simulink model "FlowControllerPrototyping"  (R2021a)
settings: Solver=VariableStepAuto  StartTime=0.0  StopTime=4  RelTol=1e-3
libraries: EdgesLibrary x8, StreetLanesLibrary x6, SourcesAndSinksLibrary x4
(part 1 of 2)
settings Model: Creator=phill  LastModifiedBy=phill

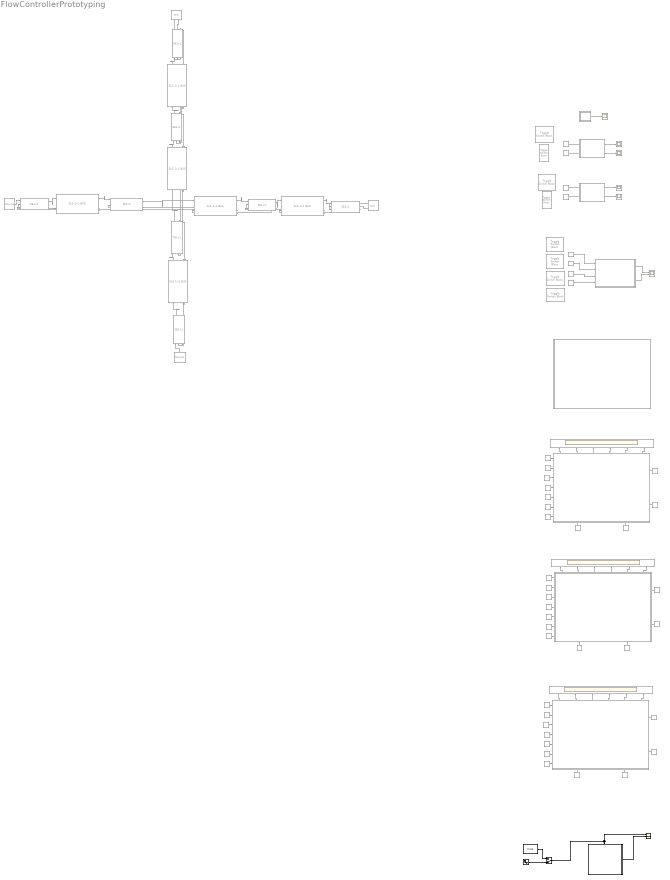
== system FlowControllerPrototyping ==
  note: Test if we can use input events to activate our controllers only if some of the inputs change. Result: Regardless of what the input event is set to (rising/falling/both), it CONSISTENTLY misses to trigger on the first of the afronementioned occurences
  note: does not work completely
  note: Just view a conflict based purely on signal strength ("car is waiting at signalX"),
      | without asking for the filling state of cross-section-segments. In this case
      | signal1 has priority before signal2
  note: Test: see how we can execute multiple transitions inside the chart during a single outer simulation step. seems to work if we chain the transitions after another using junctions
  note: does not work completely
  note: does not work completely
  note: seems to work
  Ali : Constant  Commented=on
  Ali Bo : Constant  Commented=on  Value=0
  Ali Bo1 : Constant  Commented=on  Value=0
  Ali Bo2 : Constant  Commented=on  Value=0
  Ali1 : Constant  Commented=on
  Ali2 : Constant  Commented=on
  Ari : Constant  Commented=on
  Ari Co : Constant  Commented=on  Value=0
  Ari Co1 : Constant  Commented=on  Value=0
  Ari Co2 : Constant  Commented=on  Value=0
  Ari1 : Constant  Commented=on
  Ari2 : Constant  Commented=on
  Brs : Constant  Commented=on
  Brs Ao : Constant  Commented=on  Value=0
  Brs Ao1 : Constant  Commented=on  Value=0
  Brs Ao2 : Constant  Commented=on  Value=0
  Brs Co : Constant  Commented=on
  Brs Co1 : Constant  Commented=on  Value=0
  Brs Co2 : Constant  Commented=on  Value=0
  Brs1 : Constant  Commented=on  Value=0
  Brs2 : Constant  Commented=on  Value=0
  Chart : Stateflow chart  Commented=on  TreatAsAtomicUnit=on
  Chart1 : Stateflow chart  Commented=on  TreatAsAtomicUnit=on
      settings: PortSchema="{\"entries\":[{\"content\":{\"sides\":[{\"content\":{\"connectorIds\":[\"In6\",\"In7\",\"In8\",\"In9\",\"In10\",\"In11\",\"In5\"]},\"type\":\"ConnectorPlacement.EquallySpacedRectSide\",\"uuid\":\"dee1a780-e9dd-4205-adb9-3e9cb1ec0cd6\"},{\"content\":{\"connectorIds\":[\"In4\",\"In3\"],\"side\":\"RIGHT\"},\"type\":\"ConnectorPlacement.EquallySpacedRectSide\",\"uuid\":\"bc6af08d-2df8-4a74-93d0-032b7c1c381c\"},{\"content\":{\"connectorIds\":[\"Out5\",\"Out6\",\"Out1\",\"Out2\",\"Out3\",\"Out4\"],\"side\":\"TOP\"},\"type\":\"ConnectorPlacement.EquallySpacedRectSide\",\"uuid\":\"98fea325-c9fc-472d-8e1a-d846d6e99e12\"},{\"content\":{\"connectorIds\":[\"In1\",\"In2\"],\"side\":\"BOTTOM\"},\"type\":\"ConnectorPlacement.EquallySpacedRectSide\",\"uuid\":\"a092283f-ef46-48e2-a5f8-8210ac00b2f9\"}]},\"type\":\"ConnectorPlacement.EquallySpacedConnector\",\"uuid\":\"33a851aa-4180-41c0-b4bb-9b9c3be41936\"}],\"packageUris\":[\"http://schema.mathworks.com/mf0/Connector/R2020b\"],\"version\":\"1.0\"}"
  Chart2 : Stateflow chart  Commented=on  TreatAsAtomicUnit=on
      settings: PortSchema="{\"entries\":[{\"content\":{\"sides\":[{\"content\":{\"connectorIds\":[\"In6\",\"In7\",\"In8\",\"In9\",\"In10\",\"In11\",\"In5\"]},\"type\":\"ConnectorPlacement.EquallySpacedRectSide\",\"uuid\":\"dee1a780-e9dd-4205-adb9-3e9cb1ec0cd6\"},{\"content\":{\"connectorIds\":[\"In4\",\"In3\"],\"side\":\"RIGHT\"},\"type\":\"ConnectorPlacement.EquallySpacedRectSide\",\"uuid\":\"bc6af08d-2df8-4a74-93d0-032b7c1c381c\"},{\"content\":{\"connectorIds\":[\"Out5\",\"Out6\",\"Out1\",\"Out2\",\"Out3\",\"Out4\"],\"side\":\"TOP\"},\"type\":\"ConnectorPlacement.EquallySpacedRectSide\",\"uuid\":\"98fea325-c9fc-472d-8e1a-d846d6e99e12\"},{\"content\":{\"connectorIds\":[\"In1\",\"In2\"],\"side\":\"BOTTOM\"},\"type\":\"ConnectorPlacement.EquallySpacedRectSide\",\"uuid\":\"a092283f-ef46-48e2-a5f8-8210ac00b2f9\"}]},\"type\":\"ConnectorPlacement.EquallySpacedConnector\",\"uuid\":\"33a851aa-4180-41c0-b4bb-9b9c3be41936\"}],\"packageUris\":[\"http://schema.mathworks.com/mf0/Connector/R2020b\"],\"version\":\"1.0\"}"
  Chart3 : Stateflow chart  Commented=on  TreatAsAtomicUnit=on
      settings: PortSchema="{\"entries\":[{\"content\":{\"sides\":[{\"content\":{\"connectorIds\":[\"In6\",\"In7\",\"In8\",\"In9\",\"In10\",\"In11\",\"In5\"]},\"type\":\"ConnectorPlacement.EquallySpacedRectSide\",\"uuid\":\"dee1a780-e9dd-4205-adb9-3e9cb1ec0cd6\"},{\"content\":{\"connectorIds\":[\"In4\",\"In3\"],\"side\":\"RIGHT\"},\"type\":\"ConnectorPlacement.EquallySpacedRectSide\",\"uuid\":\"bc6af08d-2df8-4a74-93d0-032b7c1c381c\"},{\"content\":{\"connectorIds\":[\"Out5\",\"Out6\",\"Out1\",\"Out2\",\"Out3\",\"Out4\"],\"side\":\"TOP\"},\"type\":\"ConnectorPlacement.EquallySpacedRectSide\",\"uuid\":\"98fea325-c9fc-472d-8e1a-d846d6e99e12\"},{\"content\":{\"connectorIds\":[\"In1\",\"In2\"],\"side\":\"BOTTOM\"},\"type\":\"ConnectorPlacement.EquallySpacedRectSide\",\"uuid\":\"a092283f-ef46-48e2-a5f8-8210ac00b2f9\"}]},\"type\":\"ConnectorPlacement.EquallySpacedConnector\",\"uuid\":\"33a851aa-4180-41c0-b4bb-9b9c3be41936\"}],\"packageUris\":[\"http://schema.mathworks.com/mf0/Connector/R2020b\"],\"version\":\"1.0\"}"
  Chart4 : Stateflow chart  Commented=on  TreatAsAtomicUnit=on
      settings: PortSchema="{\"entries\":[{\"content\":{\"sides\":[{\"content\":{\"connectorIds\":[\"In6\",\"In7\",\"In8\",\"In9\",\"In10\",\"In11\",\"In5\"]},\"type\":\"ConnectorPlacement.EquallySpacedRectSide\",\"uuid\":\"dee1a780-e9dd-4205-adb9-3e9cb1ec0cd6\"},{\"content\":{\"connectorIds\":[\"In4\",\"In3\"],\"side\":\"RIGHT\"},\"type\":\"ConnectorPlacement.EquallySpacedRectSide\",\"uuid\":\"bc6af08d-2df8-4a74-93d0-032b7c1c381c\"},{\"content\":{\"connectorIds\":[\"Out5\",\"Out6\",\"Out1\",\"Out2\",\"Out3\",\"Out4\"],\"side\":\"TOP\"},\"type\":\"ConnectorPlacement.EquallySpacedRectSide\",\"uuid\":\"98fea325-c9fc-472d-8e1a-d846d6e99e12\"},{\"content\":{\"connectorIds\":[\"In1\",\"In2\"],\"side\":\"BOTTOM\"},\"type\":\"ConnectorPlacement.EquallySpacedRectSide\",\"uuid\":\"a092283f-ef46-48e2-a5f8-8210ac00b2f9\"}]},\"type\":\"ConnectorPlacement.EquallySpacedConnector\",\"uuid\":\"33a851aa-4180-41c0-b4bb-9b9c3be41936\"}],\"packageUris\":[\"http://schema.mathworks.com/mf0/Connector/R2020b\"],\"version\":\"1.0\"}"
  Cl : Constant  Commented=on
  Cl Ao : Constant  Commented=on  Value=0
  Cl Ao1 : Constant  Commented=on  Value=0
  Cl Ao2 : Constant  Commented=on  Value=0
  Cl1 : Constant  Commented=on
  Cl2 : Constant  Commented=on
  Cs : Constant  Commented=on  Value=0
  Cs Bo : Constant  Commented=on  Value=0
  Cs Bo1 : Constant  Commented=on  Value=0
  Cs Bo2 : Constant  Commented=on  Value=0
  Cs1 : Constant  Commented=on  Value=0
  Cs2 : Constant  Commented=on  Value=0
  Manual Switch : ManualSwitch  CurrentSetting=0
  Pulse Generator : DiscretePulseGenerator  PulseType=Time based  Period=1  PulseWidth=50  PhaseDelay=1
  SE1x{1..6} (6 alike) : EdgesLibrary/SE1x1  Commented=on  Rk=1
  SLS 1x1 BUS{,1..5} (6 alike) : StreetLanesLibrary/SLS 1x1 BUS  Commented=on  Kz=3  Tz=1
  Scope{,1..4} (5 alike) : Scope  Commented=on
  Scope5 : Scope  Commented=on  NumInputPorts=2
  Scope6 : Scope  Commented=on  NumInputPorts=6
  Scope7 : Scope  Commented=on  NumInputPorts=6
  Scope8 : Scope  Commented=on  NumInputPorts=6
  Scope9 : Scope  NumInputPorts=2
  SimpleFlowController : Stateflow chart  Commented=on  TreatAsAtomicUnit=on
  Sine Wave : Sin  SampleTime=0
  Sink : SourcesAndSinksLibrary/Sink  Commented=on  SystemSampleTime=-1  VariantActivationTime=update diagram  Latency=0  AutoFrameSizeCalculation=off
      settings: PortSchema="{\"entries\":[{\"content\":{\"sides\":[{\"content\":{\"connectorIds\":[\"Out1\",\"Out2\"]},\"type\":\"ConnectorPlacement.EquallySpacedRectSide\",\"uuid\":\"9fd2383e-3590-4f0f-bafc-5a4adfbb32b4\"},{\"content\":{\"connectorIds\":[],\"side\":\"RIGHT\"},\"type\":\"ConnectorPlacement.EquallySpacedRectSide\",\"uuid\":\"1e687aa9-1098-45bd-a1f6-ea403f3f2897\"},{\"content\":{\"connectorIds\":[],\"side\":\"TOP\"},\"type\":\"ConnectorPlacement.EquallySpacedRectSide\",\"uuid\":\"fe6eaa71-085c-414b-983a-a0e72e52a49c\"}]},\"type\":\"ConnectorPlacement.EquallySpacedConnector\",\"uuid\":\"370c1712-4373-4726-99c2-6cb04807ece1\"}],\"packageUris\":[\"http://schema.mathworks.com/mf0/Connector/R2020b\"],\"version\":\"1.0\"}"
  Sink1 : SourcesAndSinksLibrary/Sink  Commented=on  SystemSampleTime=-1  VariantActivationTime=update diagram  Latency=0  AutoFrameSizeCalculation=off
      settings: PortSchema="{\"entries\":[{\"content\":{\"sides\":[{\"content\":{\"connectorIds\":[\"Out1\",\"Out2\"]},\"type\":\"ConnectorPlacement.EquallySpacedRectSide\",\"uuid\":\"9fd2383e-3590-4f0f-bafc-5a4adfbb32b4\"},{\"content\":{\"connectorIds\":[],\"side\":\"RIGHT\"},\"type\":\"ConnectorPlacement.EquallySpacedRectSide\",\"uuid\":\"1e687aa9-1098-45bd-a1f6-ea403f3f2897\"},{\"content\":{\"connectorIds\":[],\"side\":\"TOP\"},\"type\":\"ConnectorPlacement.EquallySpacedRectSide\",\"uuid\":\"fe6eaa71-085c-414b-983a-a0e72e52a49c\"}]},\"type\":\"ConnectorPlacement.EquallySpacedConnector\",\"uuid\":\"370c1712-4373-4726-99c2-6cb04807ece1\"}],\"packageUris\":[\"http://schema.mathworks.com/mf0/Connector/R2020b\"],\"version\":\"1.0\"}"
  Source : SourcesAndSinksLibrary/Source  Commented=on  SystemSampleTime=-1  VariantActivationTime=update diagram  Latency=0  AutoFrameSizeCalculation=off
  Source1 : SourcesAndSinksLibrary/Source  Commented=on  SystemSampleTime=-1  VariantActivationTime=update diagram  Latency=0  AutoFrameSizeCalculation=off
  TE1x1 : EdgesLibrary/TE1x1  Commented=on  Rk=1
  TE1x2 : EdgesLibrary/TE1x1  Commented=on  Rk=1
  Testchart : Stateflow chart  TreatAsAtomicUnit=on
  Toggle Switch{,1..7} (8 alike) : ToggleSwitchBlock  Commented=on
      settings: Values={{'Off', 'On'}, [0 1]}
  innerBT : Constant  Commented=on  Value=0
  innerLR : Constant  Commented=on  Value=0
  mincontroller_pseudoparallel : Stateflow chart  Commented=on  TreatAsAtomicUnit=on
  mincontroller_sequential : Stateflow chart  Commented=on  TreatAsAtomicUnit=on
  x01 : Constant  Commented=on
  x02 : Constant  Commented=on
  x0Bottom : Constant  Commented=on
  x0Left : Constant  Commented=on
  x0a : Constant  Commented=on
  x0b : Constant  Commented=on
  wires:
  Source/1 -> SE1x4/1
  SLS 1x1 BUS/6 -> SE1x4/2
  SLS 1x1 BUS/7 -> SE1x4/3
  SE1x4/1 -> SLS 1x1 BUS/1
  SLS 1x1 BUS/2 -> TE1x1/1
  TE1x1/2 -> SLS 1x1 BUS/2
  SLS 1x1 BUS1/6 -> TE1x1/3
  SLS 1x1 BUS1/7 -> TE1x1/4
  TE1x1/1 -> SLS 1x1 BUS1/1
  SLS 1x1 BUS1/2 -> SE1x1/1
  SE1x1/2 -> SLS 1x1 BUS1/2
  SLS 1x1 BUS2/6 -> SE1x1/2
  SLS 1x1 BUS2/7 -> SE1x1/3
  SE1x1/1 -> SLS 1x1 BUS2/1
  SLS 1x1 BUS2/2 -> SE1x3/1
  SE1x3/2 -> SLS 1x1 BUS2/2
  Sink/1 -> SE1x3/2
  Sink/2 -> SE1x3/3
  Source1/1 -> SE1x5/1
  SE1x5/1 -> SLS 1x1 BUS3/1
  SLS 1x1 BUS3/6 -> SE1x5/2
  SLS 1x1 BUS3/7 -> SE1x5/3
  TE1x2/2 -> SLS 1x1 BUS3/2
  SLS 1x1 BUS3/2 -> TE1x2/1
  TE1x2/1 -> SLS 1x1 BUS4/1
  SLS 1x1 BUS4/7 -> TE1x2/4
  SLS 1x1 BUS4/6 -> TE1x2/3
  SE1x2/2 -> SLS 1x1 BUS4/2
  SLS 1x1 BUS4/2 -> SE1x2/1
  SE1x2/1 -> SLS 1x1 BUS5/1
  SLS 1x1 BUS5/7 -> SE1x2/3
  SLS 1x1 BUS5/6 -> SE1x2/2
  SE1x6/2 -> SLS 1x1 BUS5/2
  SLS 1x1 BUS5/2 -> SE1x6/1
  Sink1/1 -> SE1x6/2
  Sink1/2 -> SE1x6/3
  Chart/1(y) -> Scope/1
  x01/1 -> mincontroller_pseudoparallel/1(signal1)
  x02/1 -> mincontroller_pseudoparallel/2(signal2)
  mincontroller_pseudoparallel/1(enable1) -> Scope1/1
  mincontroller_pseudoparallel/2(enable2) -> Scope2/1
  mincontroller_sequential/1(enable1) -> Scope3/1
  mincontroller_sequential/2(enable2) -> Scope4/1
  x0a/1 -> mincontroller_sequential/1(signal1)
  x0b/1 -> mincontroller_sequential/2(signal2)
  x0Left/1 -> SimpleFlowController/1(x0Left)
  x0Bottom/1 -> SimpleFlowController/2(x0Bottom)
  innerLR/1 -> SimpleFlowController/3(innerLR)
  innerBT/1 -> SimpleFlowController/4(innerBT)
  SimpleFlowController/1(openLeft) -> Scope5/1
  SimpleFlowController/2(openBottom) -> Scope5/2
  Ali Bo/1 -> Chart2/6(Ali_Bo)
  Ari Co/1 -> Chart2/7(Ari_Co)
  Ali/1 -> Chart2/1(Ali)
  Ari/1 -> Chart2/2(Ari)
  Cl Ao/1 -> Chart2/8(Cl_Ao)
  Cs Bo/1 -> Chart2/9(Cs_Bo)
  Brs Co/1 -> Chart2/10(Brs_Co)
  Brs Ao/1 -> Chart2/11(Brs_Ao)
  Brs/1 -> Chart2/5(Brs)
  Chart2/5(enableBrs11) -> Scope6/1
  Chart2/6(enableBrs12) -> Scope6/2
  Chart2/1(enableAli3) -> Scope6/3
  Chart2/2(enableAri4) -> Scope6/4
  Chart2/3(enableCl7) -> Scope6/5
  Chart2/4(enableCs8) -> Scope6/6
  Cs/1 -> Chart2/4(Cs)
  Cl/1 -> Chart2/3(Cl)
  Cs1/1 -> Chart3/4(Cs)
  Cl1/1 -> Chart3/3(Cl)
  Cl Ao1/1 -> Chart3/8(Cl_Ao)
  Ari Co1/1 -> Chart3/7(Ari_Co)
  Chart3/2(enableAri4) -> Scope7/4
  Chart3/3(enableCl7) -> Scope7/5
  Ali Bo1/1 -> Chart3/6(Ali_Bo)
  Chart3/1(enableAli3) -> Scope7/3
  Chart3/6(enableBrs12) -> Scope7/2
  Cs Bo1/1 -> Chart3/9(Cs_Bo)
  Brs Co1/1 -> Chart3/10(Brs_Co)
  Chart3/4(enableCs8) -> Scope7/6
  Ali1/1 -> Chart3/1(Ali)
  Chart3/5(enableBrs11) -> Scope7/1
  Ari1/1 -> Chart3/2(Ari)
  Brs Ao1/1 -> Chart3/11(Brs_Ao)
  Brs1/1 -> Chart3/5(Brs)
  Brs2/1 -> Chart4/5(Brs)
  Chart4/3(enableCl7) -> Scope8/5
  Ali2/1 -> Chart4/1(Ali)
  Chart4/5(enableBrs11) -> Scope8/1
  Brs Ao2/1 -> Chart4/11(Brs_Ao)
  Chart4/6(enableBrs12) -> Scope8/2
  Cs Bo2/1 -> Chart4/9(Cs_Bo)
  Chart4/2(enableAri4) -> Scope8/4
  Chart4/4(enableCs8) -> Scope8/6
  Ari2/1 -> Chart4/2(Ari)
  Ali Bo2/1 -> Chart4/6(Ali_Bo)
  Cs2/1 -> Chart4/4(Cs)
  Ari Co2/1 -> Chart4/7(Ari_Co)
  Chart4/1(enableAli3) -> Scope8/3
  Cl Ao2/1 -> Chart4/8(Cl_Ao)
  Cl2/1 -> Chart4/3(Cl)
  Brs Co2/1 -> Chart4/10(Brs_Co)
  Manual Switch/1 -> Scope9/1, Testchart/Trigger
  Testchart/1(y) -> Scope9/2
  Sine Wave/1 -> Manual Switch/2
  Pulse Generator/1 -> Manual Switch/1

== stateflow chart FlowControllerPrototyping/SimpleFlowController ==
  state Initial
  note: Bottom
  note: Left
  (default) -> Initial : {openLeft = 0; openBottom = 0;}
  (junction 10) -> (junction 14) [order 1] : [x0Left > 0 && x0Bottom == 0 && innerBT == 0]{openLeft=1;}
  Initial -> (junction 10) [order 1] : [x0Bottom > 0 && innerLR == 0]{openBottom=1;}
  (junction 10) -> (junction 14) [order 2] : {openLeft=0;}
  Initial -> (junction 10) [order 2] : {openBottom=0;}
  (junction 14) -> (junction 15)
  (junction 15) -> Initial
  data: x0Left input; x0Bottom input; openLeft output; openBottom output; innerLR input; innerBT input

== stateflow chart FlowControllerPrototyping/mincontroller_sequential ==
  note: for signal 2
  note: for signal 1
  state Superstate
  (default) -> Superstate : {enable1 = 0; enable2 = 0}
  (junction 26) -> (junction 27) [order 1] : [signal2 > 0 && signal1 == 0]{enable2=1;}
  Superstate -> (junction 26) [order 1] : [signal1 > 0]{enable1 = 1;}
  Superstate -> (junction 26) [order 2] : {enable1=0;}
  (junction 26) -> (junction 27) [order 2] : {enable2=0;}
  (junction 27) -> (junction 34)
  (junction 34) -> Superstate
  data: enable1 output; enable2 output; signal1 input; signal2 input

== stateflow chart FlowControllerPrototyping/Chart1 ==
  note: Notizen (mal auf Deutsch):
      | wenn an einer kante etwas anliegt und keine der stärkeren kanten etwas anliegen hat,
      | 	und die konfliktbereiche frei sind: schalte kante frei
      | 	<Ali 3> wird dominiert von <Cl 7> und <Cs 8>  [Kreuzungen: <Brs Co> <Cl Ao> <Cs Bo>
      | 	<Ari 4> wird nicht dominiert [Kreuzungen: <Brs Co>
      | 	<Cl 7> wird dominiert von <Brs 11> und <Brs 12> [Kreuzungen: <Brs Co> <Brs Ao>
      | 	<Cs 8> wird nicht dominiert [Kreuzungen: <Ali Bo>
      | 	<Brs 11> wird dominiert von <Ali 3> und <Ari 4> [Kreuzungen: <Brs Ao> <Ali Bo> <Ari Co>
      | 	<Brs 12> wird nicht dominiert [Kreuzungen: <Cl Ao>
      |
      | 	Anmerkung: die einflüsse Brs11 und Brs12 behindern sich nicht. da beide kanten an
      | 	EIN UND DEMSELBEN SEGMENT liegen, und unsere 0.5:0.5 gewichtung schon suggeriert,
      | 	dass sich hier die autos "spalten", können sich die autos beim "Parallelen" fließen
      | 	in die segmente <Brs Co> und <Brs Ao> nicht wirklich in die quere kommen. Oder selbst wenn sie es
      |       tun, können wir nichts dagegen unternehmen - wenn wir einem der pfade gegenüber dem anderen
      | 	priorität geben, wird bei dem anderen jeweils NIE etwas fließen. Damit müssen wir wohl leben :(
      |
      | a)
      | [Ali > 0 && Cl == 0 && Cs == 0 && Brs_Co == 0 && Cl_Ao == 0 && Cs_Bo == 0]{enableAli3=1;}
      | else {enableAli3=0;}
      | b)
      | [Ari > 0 && Brs_Co == 0]{enableAri4=1;}
      | else {enableAri4=0;}
      | c)
      | [Cl > 0 && Brs == 0 && Brs_Co == 0 && Brs_Ao == 0]{enableCl7=1;}
      | else {enableCl7=0;}
      | d)
      | [Cs > 0 && Ali_Bo == 0]{enableCs8=1;}
      | else {enableCs8=0;}
      | e)
      | [Brs > 0 && Ali == 0 && Ari == 0 && Ali_Bo == 0 && Ari_Co == 0]{enableBrs11=1;}
      | else {enableBrs11=0;}
      | f)
      | [Brs > 0 && Cl_Ao == 0]{enableBrs12=1;}
      | else {enableBrs12=0;}
      |
      | Anmerkung: Da es im Falle [Ali > 0 && Brs > 0 && Cl > 0] einen deadlock gibt, müssen wir uns entscheiden, wer fahren darf. Da die "gerade" strecke vermutlich am ehesten einer hauptstraße
      | entsprechen würde, wird hier die regel so modifiziert, dass die von "unten" (Ali) kommenden autos
      | freiwillig auf Brs (und gezwungenermaßen auf Cl) warten, um stau auf der hauptstraße zu reduzieren.
      | Dazu erweitern wir die anliege-conditionen der Regel e) zu:
      | e')
      | [ ( (Brs > 0 && Ali == 0 && Ari == 0) || (Ali > 0 && Brs > 0 && Cl >0 && Ari == 0) ) && Ali_Bo == 0 && Ari_Co == 0]{enableBrs11=1;}
      | else {enableBrs11=0;} klappt nicht
      |
      | Somit verhält sich das T stück dann so, als würde magischerweise ein Vorfahrt achten schild
      | am unteren Eingang solange stehen, wie ein deadlock droht, und danach wieder verschwinden.
      | Unsere Autofahrer sind also sehr sozial unterwegs...
  note: ?
  state InitiatePerStepCheck
  note: Brs-11-<Brs Co>-6-Co
      | (Links will geradeaus)
  note: Brs-12-<Brs Ao>-1-Ao
      | (Links will geradeaus)
  note: Ari-4-<Ari Co>-5-Co
      | (Unten will rechts abbiegen)
  note: Cl-7-<Cl Ao>-2-Ao
      | (Rechts will links abbiegen)
  note: Cs-8-<Cl Ao>-9-Bo
      | (Rechts will geradeaus)
  note: Ali-3-<Ali Bo>-10-Bo
      | (Unten will Links abbiegen)
  note: Deadlock-Resolution
  InitiatePerStepCheck -> (junction 23) [order 1] : [Ali > 0 && Cl == 0 && Cs == 0 && Brs_Co == 0 && Cl_Ao == 0 && Cs_Bo == 0]
      | {enableAli3=1;}
  (junction 23) -> (junction 29) [order 1] : [Ari > 0 && Brs_Co == 0]{enableAri4=1;}
  (junction 29) -> (junction 36) [order 1] : [Cl > 0 && Brs == 0 && Brs_Co == 0 && Brs_Ao == 0]{enableCl7=1; }
  (junction 39) -> (junction 40) [order 1] : [  ( (Brs > 0 && Ali == 0 && Ari == 0) || (Ali > 0 && Brs > 0 && Cl > 0 && Ari == 0) ) && Ali_Bo == 0 && Ari_Co == 0]{enableBrs11=1;}
  (junction 40) -> (junction 45) [order 1] : [Brs > 0 && Cl_Ao == 0]{enableBrs12=1;}
  (junction 36) -> (junction 39) [order 1] : [Cs > 0 && Ali_Bo == 0]{enableCs8=1;}
  (junction 39) -> (junction 40) [order 2] : {enableBrs11=0;}
  (junction 29) -> (junction 36) [order 2] : {enableCl7=0;}
  (junction 36) -> (junction 39) [order 2] : {enableCs8=0;}
  (junction 23) -> (junction 29) [order 2] : {enableAri4=0;}
  (junction 40) -> (junction 45) [order 2] : {enableBrs12=0;}
  InitiatePerStepCheck -> (junction 23) [order 2] : {enableAli3=0;}
  (junction 45) -> (junction 53)
  (default) -> InitiatePerStepCheck : {enableAli3 = 0; enableAri4 = 0;
      | enableCl7 = 0; enableCs8 = 0;
      | enableBrs11 = 0; enableBrs12 = 0;}
  (junction 53) -> InitiatePerStepCheck
  data: Ali input; Ari input; Cl input; Cs input; Brs input; Ali_Bo input; Ari_Co input; Cl_Ao input; Cs_Bo input; Brs_Co input; Brs_Ao input; enableAli3 output; enableAri4 output; enableCl7 output; enableCs8 output; enableBrs11 output; enableBrs12 output

== stateflow chart FlowControllerPrototyping/Chart2 ==
  note: Notizen (mal auf Deutsch):
      | wenn an einer kante etwas anliegt und keine der stärkeren kanten etwas anliegen hat,
      | 	und die konfliktbereiche frei sind: schalte kante frei
      | 	<Ali 3> wird dominiert von <Cl 7> und <Cs 8>  [Kreuzungen: <Brs Co> <Cl Ao> <Cs Bo>
      | 	<Ari 4> wird nicht dominiert [Kreuzungen: <Brs Co>
      | 	<Cl 7> wird dominiert von <Brs 11> und <Brs 12> [Kreuzungen: <Brs Co> <Brs Ao>
      | 	<Cs 8> wird nicht dominiert [Kreuzungen: <Ali Bo>
      | 	<Brs 11> wird dominiert von <Ali 3> und <Ari 4> [Kreuzungen: <Brs Ao> <Ali Bo> <Ari Co>
      | 	<Brs 12> wird nicht dominiert [Kreuzungen: <Cl Ao>
      |
      | 	Anmerkung: die einflüsse Brs11 und Brs12 behindern sich nicht. da beide kanten an
      | 	EIN UND DEMSELBEN SEGMENT liegen, und unsere 0.5:0.5 gewichtung schon suggeriert,
      | 	dass sich hier die autos "spalten", können sich die autos beim "Parallelen" fließen
      | 	in die segmente <Brs Co> und <Brs Ao> nicht wirklich in die quere kommen. Oder selbst wenn sie es
      |       tun, können wir nichts dagegen unternehmen - wenn wir einem der pfade gegenüber dem anderen
      | 	priorität geben, wird bei dem anderen jeweils NIE etwas fließen. Damit müssen wir wohl leben :(
      |
      | a)
      | [Ali > 0 && Cl == 0 && Cs == 0 && Brs_Co == 0 && Cl_Ao == 0 && Cs_Bo == 0]{enableAli3=1;}
      | else {enableAli3=0;}
      | b)
      | [Ari > 0 && Brs_Co == 0]{enableAri4=1;}
      | else {enableAri4=0;}
      | c)
      | [Cl > 0 && Brs == 0 && Brs_Co == 0 && Brs_Ao == 0]{enableCl7=1;}
      | else {enableCl7=0;}
      | d)
      | [Cs > 0 && Ali_Bo == 0]{enableCs8=1;}
      | else {enableCs8=0;}
      | e)
      | [Brs > 0 && Ali == 0 && Ari == 0 && Ali_Bo == 0 && Ari_Co == 0]{enableBrs11=1;}
      | else {enableBrs11=0;}
      | f)
      | [Brs > 0 && Cl_Ao == 0]{enableBrs12=1;}
      | else {enableBrs12=0;}
      |
      | Anmerkung: Da es im Falle [Ali > 0 && Brs > 0 && Cl > 0] einen deadlock gibt, müssen wir uns entscheiden, wer fahren darf. Da die "gerade" strecke vermutlich am ehesten einer hauptstraßeentsprechen würde, wird hier die regel so modifiziert, dass die von "unten" (Ali) kommenden autos freiwillig auf Brs (und gezwungenermaßen auf Cl) warten, um stau auf der hauptstraße zu reduzieren. Wenn Ali sein Fahrtrecht an Brs abgiebt, gibt es nun zwei Fälle zu beachten:
      | 	a ) im falle [Ari == 0] kann Brs versuchen, sich freizuschalten, da der weg frei ist
      |       b) im falle [Ari != 0] würde Brs sehen, dass eine fahrt nicht möglich ist, und stattdessen sein von Ali erhaltenes Recht
      |            an Cl weitergeben
      | Natürlich sieht der automat immer nur eine momentaufnahme, und selbst, wenn beide fälle abgefragt wurden, muss
      | nicht automatisch ein fluss garantiert sein, da sich immernoch aufgrund früherer verkehrsflüsse autos in den
      | zwischensegmenten aufhalten können, und so eine aktivierung von Ali/Brs/Cl verhindern, bis die segmente evakuiert sind.
      |
      | Hinweis: wirklich effektiv ist diese maßnahme nicht, da unsere 1-zu-2 kanten einfach die ansonsten verwendete rate halbieren, und jederzeit gleichzeitig fließen. wenn also an Brs etwas anliegt, kann Brs-12 IMMER fließen, was bedeutet, dass Cl immer warten muss. Im Falle [Ali > 0 && Brs > 0 && Cl > 0 && Ari > 0] können keine der drei eingänge 11,3,7 öffnen.
  note: ?
  state InitiatePerStepCheck
  note: Brs-11-<Brs Co>-6-Co
      | (Links will geradeaus)
  note: Brs-12-<Brs Ao>-1-Ao
      | (Links will geradeaus)
  note: Ari-4-<Ari Co>-5-Co
      | (Unten will rechts abbiegen)
  note: Cl-7-<Cl Ao>-2-Ao
      | (Rechts will links abbiegen)
  note: Cs-8-<Cl Ao>-9-Bo
      | (Rechts will geradeaus)
  note: Ali-3-<Ali Bo>-10-Bo
      | (Unten will Links abbiegen)
  note: Deadlock-Detection
  note: Deadlock-Resolution
  InitiatePerStepCheck -> (junction 23) [order 1] : [Ali > 0 && Cl == 0 && Cs == 0 && Brs_Co == 0 && Cl_Ao == 0 && Cs_Bo == 0]
      | {enableAli3=1; }
  (junction 23) -> (junction 29) [order 1] : [Ari > 0 && Brs_Co == 0]{enableAri4=1;}
  (junction 29) -> (junction 36) [order 1] : [Cl > 0 && Brs == 0 && Brs_Co == 0 && Brs_Ao == 0]{enableCl7=1; }
  (junction 39) -> (junction 40) [order 1] : [Brs > 0 && Ali == 0 && Ari == 0 && Ali_Bo == 0 && Ari_Co == 0]{enableBrs11=1;}
  (junction 40) -> (junction 45) [order 1] : [Brs > 0 && Cl_Ao == 0]{enableBrs12=1;}
  (junction 36) -> (junction 39) [order 1] : [Cs > 0 && Ali_Bo == 0]{enableCs8=1;}
  (junction 39) -> (junction 40) [order 2] : {enableBrs11=0;}
  (junction 29) -> (junction 36) [order 2] : {enableCl7=0;}
  (junction 36) -> (junction 39) [order 2] : {enableCs8=0;}
  (junction 23) -> (junction 29) [order 2] : {enableAri4=0;}
  (junction 40) -> (junction 45) [order 2] : {enableBrs12=0;}
  InitiatePerStepCheck -> (junction 23) [order 2] : {enableAli3=0;}
  (junction 45) -> (junction 53)
  (junction 53) -> InitiatePerStepCheck [order 2]
  (junction 53) -> (junction 64) [order 1] : [Ali > 0 && Brs > 0 && Cl > 0]
  (default) -> InitiatePerStepCheck : {enableAli3 = 0; enableAri4 = 0;
      | enableCl7 = 0; enableCs8 = 0;
      | enableBrs11 = 0; enableBrs12 = 0;}
  (junction 67) -> (junction 71) [order 1] : [Brs_Co == 0 && Brs_Ao == 0]{enableCl7=1;}
  (junction 64) -> (junction 67) [order 1] : [Ari > 0]
  (junction 64) -> (junction 69) [order 2]
  (junction 67) -> (junction 71) [order 2]
  (junction 71) -> InitiatePerStepCheck
  (junction 69) -> (junction 71) [order 2]
  (junction 69) -> (junction 71) [order 1] : [Ali_Bo == 0 && Ari_Co == 0]{enableBrs11=1;}
  data: Ali input; Ari input; Cl input; Cs input; Brs input; Ali_Bo input; Ari_Co input; Cl_Ao input; Cs_Bo input; Brs_Co input; Brs_Ao input; enableAli3 output; enableAri4 output; enableCl7 output; enableCs8 output; enableBrs11 output; enableBrs12 output

== stateflow chart FlowControllerPrototyping/Chart3 ==
  note: Notizen (mal auf Deutsch):
      | wenn an einer kante etwas anliegt und keine der stärkeren kanten etwas anliegen hat,
      | 	und die konfliktbereiche frei sind: schalte kante frei
      | 	<Ali 3> wird dominiert von <Cl 7> und <Cs 8>  [Kreuzungen: <Brs Co> <Cl Ao> <Cs Bo>
      | 	<Ari 4> wird nicht dominiert [Kreuzungen: <Brs Co>
      | 	<Cl 7> wird dominiert von <Brs 11> und <Brs 12> [Kreuzungen: <Brs Co> <Brs Ao>
      | 	<Cs 8> wird nicht dominiert [Kreuzungen: <Ali Bo>
      | 	<Brs 11> wird dominiert von <Ali 3> und <Ari 4> [Kreuzungen: <Brs Ao> <Ali Bo> <Ari Co>
      | 	<Brs 12> wird nicht dominiert [Kreuzungen: <Cl Ao>
      |
      | 	Anmerkung: die einflüsse Brs11 und Brs12 behindern sich nicht. da beide kanten an
      | 	EIN UND DEMSELBEN SEGMENT liegen, und unsere 0.5:0.5 gewichtung schon suggeriert,
      | 	dass sich hier die autos "spalten", können sich die autos beim "Parallelen" fließen
      | 	in die segmente <Brs Co> und <Brs Ao> nicht wirklich in die quere kommen. Oder selbst wenn sie es
      |       tun, können wir nichts dagegen unternehmen - wenn wir einem der pfade gegenüber dem anderen
      | 	priorität geben, wird bei dem anderen jeweils NIE etwas fließen. Damit müssen wir wohl leben :(
      |
      | a)
      | if [Ali > 0 && Cl == 0 && Cs == 0 && Brs_Co == 0 && Cl_Ao == 0 && Cs_Bo == 0]{enableAli3=1;}
      | else {enableAli3=0;}
      | b)
      | if [Ari > 0 && Brs_Co == 0]{enableAri4=1;}
      | else {enableAri4=0;}
      | c)
      | if [Cl > 0 && Brs == 0 && Brs_Co == 0 && Brs_Ao == 0]{enableCl7=1;}
      | else {enableCl7=0;}
      | d)
      | if [Cs > 0 && Ali_Bo == 0]{enableCs8=1;}
      | else {enableCs8=0;}
      | e)
      | if [Brs > 0 && Ali == 0 && Ari == 0 && Ali_Bo == 0 && Ari_Co == 0]{enableBrs11=1;}
      | else {enableBrs11=0;}
      | f)
      | if [Brs > 0 && Cl_Ao == 0]{enableBrs12=1;}
      | else {enableBrs12=0;}
      |
      | Anmerkung: Da es im Falle [Ali > 0 && Brs > 0 && Cl > 0] einen deadlock gibt, müssen wir uns entscheiden, wer fahren darf.
      |
      | // Brs11 soll das fahrtrecht bekommen, um den fluss entlang der geraden aufrechtzuerhalten, wenn möglich
      | if [Ari == 0 && (Ari_Co == 0 && Ali_Bo == 0){enableBrs11=1;}
      | else
      |
      |       // falls Brs12 nicht kann, versucht Ali zu fahren. Eigentlich müsste Cl die nächstbeste Wahl sein,
      | 	// allerdings kann Cl im falle eines Deadlocks ohnehin nicht fließen, da wegen unserer modellierung
      | 	// der 1x2 kanten (bzw. 1x2 segmente) gilt "Deadlock => [Brs > 0] => [Brs12 will aktiv sein]" - und da
      |       // Brs12 vorrang vor Cl7 hat, ist Cl7 in diesem szenario grundsätzlich blockiert.
      | 	if [Cs == 0 && (Brs_Co == 0 && Cl_Ao == 0 && Cs_Bo == 0)]{enableAli3=1;}
      | 	else //guess noone can make it
  note: ?
  state InitiatePerStepCheck
  note: Brs-11-<Brs Co>-6-Co
      | (Links will geradeaus)
  note: Brs-12-<Brs Ao>-1-Ao
      | (Links will geradeaus)
  note: Ari-4-<Ari Co>-5-Co
      | (Unten will rechts abbiegen)
  note: Cl-7-<Cl Ao>-2-Ao
      | (Rechts will links abbiegen)
  note: Cs-8-<Cl Ao>-9-Bo
      | (Rechts will geradeaus)
  note: Ali-3-<Ali Bo>-10-Bo
      | (Unten will Links abbiegen)
  note: Deadlock-Detection
  note: Deadlock-Resolution
  note: Anstelle der ebene für deadlock resolution konnte man den "Links will geradeaus" bereich in der reihenfolge VOR "Unten will links abbiegen" setzen. "Links will geradeaus" muss dann um eine weitere kante mit höchster priorität ergänzt werden mit einem label
      | [ (Ali > 0 && Brs > 0 && Cl > 0 ) && (Ari == 0 && Ali_Bo == 0 && Ari_Co == 0]{enableBrs11=1;}
      |
      | "Unten will links abbiegen" wird dann ebenfalls um eine Kante mit höchster priorität ergänzt mit dem Label
      | [ (Ali > 0 && Brs > 0 && Cl > 0) && (Cs_Bo == 0 && Cl_Ao == 0) && ~(enableBrs11==1)
  InitiatePerStepCheck -> (junction 23) [order 1] : [Ali > 0 && Cl == 0 && Cs == 0 && Brs_Co == 0 && Cl_Ao == 0 && Cs_Bo == 0]
      | {enableAli3=1; }
  (junction 23) -> (junction 29) [order 1] : [Ari > 0 && Brs_Co == 0]{enableAri4=1;}
  (junction 29) -> (junction 36) [order 1] : [Cl > 0 && Brs == 0 && Brs_Co == 0 && Brs_Ao == 0]{enableCl7=1; }
  (junction 39) -> (junction 40) [order 1] : [Brs > 0 && Ali == 0 && Ari == 0 && Ali_Bo == 0 && Ari_Co == 0]{enableBrs11=1;}
  (junction 40) -> (junction 45) [order 1] : [Brs > 0 && Cl_Ao == 0]{enableBrs12=1;}
  (junction 36) -> (junction 39) [order 1] : [Cs > 0 && Ali_Bo == 0]{enableCs8=1;}
  (junction 39) -> (junction 40) [order 2] : {enableBrs11=0;}
  (junction 29) -> (junction 36) [order 2] : {enableCl7=0;}
  (junction 36) -> (junction 39) [order 2] : {enableCs8=0;}
  (junction 23) -> (junction 29) [order 2] : {enableAri4=0;}
  (junction 40) -> (junction 45) [order 2] : {enableBrs12=0;}
  InitiatePerStepCheck -> (junction 23) [order 2] : {enableAli3=0;}
  (junction 45) -> (junction 53)
  (junction 53) -> InitiatePerStepCheck [order 2]
  (junction 53) -> (junction 64) [order 1] : [Ali > 0 && Brs > 0 && Cl > 0]
  (default) -> InitiatePerStepCheck : {enableAli3 = 0; enableAri4 = 0;
      | enableCl7 = 0; enableCs8 = 0;
      | enableBrs11 = 0; enableBrs12 = 0;}
  (junction 64) -> (junction 71) [order 1] : [Ari == 0 && Ali_Bo == 0 && Ari_Co == 0]{enableBrs11=1;}
  (junction 64) -> (junction 71) [order 2] : [Ari > 0 && Cs == 0 && (Brs_Co == 0 && Cl_Ao == 0 && Cs_Bo == 0)]{enableAli3=1;}
  (junction 71) -> InitiatePerStepCheck
  data: Ali input; Ari input; Cl input; Cs input; Brs input; Ali_Bo input; Ari_Co input; Cl_Ao input; Cs_Bo input; Brs_Co input; Brs_Ao input; enableAli3 output; enableAri4 output; enableCl7 output; enableCs8 output; enableBrs11 output; enableBrs12 output
